simulink model "teste_amortecedor"  (R2019b)
settings: Solver=FixedStepAuto  StartTime=0.0  StopTime=10  FixedStep=10^-3  RelTol=1e-3
undefined symbols (not defined in the file or in its folder): sigbuilder_block
settings Model: Creator=aluno  LastModifiedBy=aluno

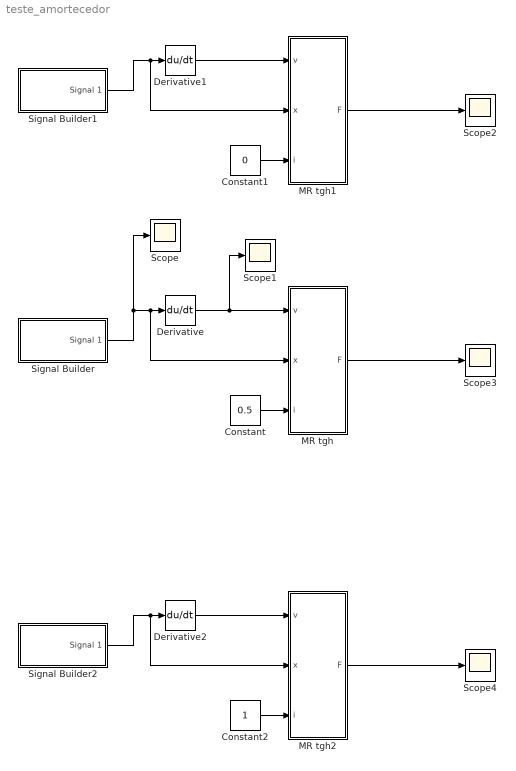
== system teste_amortecedor ==
  Constant : Constant  Value=0.5
  Constant1 : Constant  Value=0
  Constant2 : Constant
  Derivative : Derivative
  Derivative1 : Derivative
  Derivative2 : Derivative
  MR tgh : MATLAB Function  TreatAsAtomicUnit=on
  MR tgh1 : MATLAB Function  TreatAsAtomicUnit=on
  MR tgh2 : MATLAB Function  TreatAsAtomicUnit=on
  Scope{,1..4} (5 alike) : Scope
  Signal Builder : Subsystem  Tag=STV Subsys  LoadFcn=sigbuilder_block('load');  StartFcn=sigbuilder_block('start');  StopFcn=sigbuilder_block('stop');  ClipboardFcn=sigbuilder_block('clipboard');  mask(Sigbuilder block){tuvar=[0:10]}
      mask help: Simulink:masks:SigbuilderBlock_MD
      mask init:
      | if ~strcmp(get_param(bdroot(gcbh),'SimulationStatus'),'stopped') tuvar = sigbuilder_block('maskInit'); end
      settings: CopyFcn=sigbuilder_block('copy');  DeleteFcn=sigbuilder_block('delete');  ModelCloseFcn=sigbuilder_block('modelClose');  PreSaveFcn=sigbuilder_block('preSave');  PauseFcn=sigbuilder_block('pause');  ContinueFcn=sigbuilder_block('continue');  NameChangeFcn=sigbuilder_block('namechange');  OpenFcn=sigbuilder_block('open',[437.6 199.2 550.4 400 ]);  CloseFcn=sigbuilder_block('close');
      mask Display: plot(0, 0, 100, 100,[2, 2, 32, 32, 2], [68, 8, 8, 68, 68],[32, 2], [38, 38], [32, 19, 2],[53, 60, 44], [32, 17, 17, 2],[16, 16, 31, 31]);txt = getActiveGroup(gcbh);text(2, 100, txt,'verticalAlignment', 'top');
  Signal Builder1 : Subsystem  Tag=STV Subsys  LoadFcn=sigbuilder_block('load');  StartFcn=sigbuilder_block('start');  StopFcn=sigbuilder_block('stop');  ClipboardFcn=sigbuilder_block('clipboard');  mask(Sigbuilder block){tuvar=[0:10]}
      mask help: Simulink:masks:SigbuilderBlock_MD
      mask init:
      | if ~strcmp(get_param(bdroot(gcbh),'SimulationStatus'),'stopped') tuvar = sigbuilder_block('maskInit'); end
      settings: CopyFcn=sigbuilder_block('copy');  DeleteFcn=sigbuilder_block('delete');  ModelCloseFcn=sigbuilder_block('modelClose');  PreSaveFcn=sigbuilder_block('preSave');  PauseFcn=sigbuilder_block('pause');  ContinueFcn=sigbuilder_block('continue');  NameChangeFcn=sigbuilder_block('namechange');  OpenFcn=sigbuilder_block('open',[437.6 199.2 550.4 400 ]);  CloseFcn=sigbuilder_block('close');
      mask Display: plot(0, 0, 100, 100,[2, 2, 32, 32, 2], [68, 8, 8, 68, 68],[32, 2], [38, 38], [32, 19, 2],[53, 60, 44], [32, 17, 17, 2],[16, 16, 31, 31]);txt = getActiveGroup(gcbh);text(2, 100, txt,'verticalAlignment', 'top');
  Signal Builder2 : Subsystem  Tag=STV Subsys  LoadFcn=sigbuilder_block('load');  StartFcn=sigbuilder_block('start');  StopFcn=sigbuilder_block('stop');  ClipboardFcn=sigbuilder_block('clipboard');  mask(Sigbuilder block){tuvar=[0:10]}
      mask help: Simulink:masks:SigbuilderBlock_MD
      mask init:
      | if ~strcmp(get_param(bdroot(gcbh),'SimulationStatus'),'stopped') tuvar = sigbuilder_block('maskInit'); end
      settings: CopyFcn=sigbuilder_block('copy');  DeleteFcn=sigbuilder_block('delete');  ModelCloseFcn=sigbuilder_block('modelClose');  PreSaveFcn=sigbuilder_block('preSave');  PauseFcn=sigbuilder_block('pause');  ContinueFcn=sigbuilder_block('continue');  NameChangeFcn=sigbuilder_block('namechange');  OpenFcn=sigbuilder_block('open',[437.6 199.2 550.4 400 ]);  CloseFcn=sigbuilder_block('close');
      mask Display: plot(0, 0, 100, 100,[2, 2, 32, 32, 2], [68, 8, 8, 68, 68],[32, 2], [38, 38], [32, 19, 2],[53, 60, 44], [32, 17, 17, 2],[16, 16, 31, 31]);txt = getActiveGroup(gcbh);text(2, 100, txt,'verticalAlignment', 'top');
  wires:
  Constant/1 -> MR tgh/3(i)
  Signal Builder/1(Signal 1) -> Scope/1, MR tgh/2(x), Derivative/1
  Derivative/1 -> Scope1/1, MR tgh/1(v)
  MR tgh1/1(F) -> Scope2/1
  Constant1/1 -> MR tgh1/3(i)
  Signal Builder1/1(Signal 1) -> MR tgh1/2(x), Derivative1/1
  Derivative1/1 -> MR tgh1/1(v)
  Constant2/1 -> MR tgh2/3(i)
  Signal Builder2/1(Signal 1) -> MR tgh2/2(x), Derivative2/1
  Derivative2/1 -> MR tgh2/1(v)
  MR tgh/1(F) -> Scope3/1
  MR tgh2/1(F) -> Scope4/1

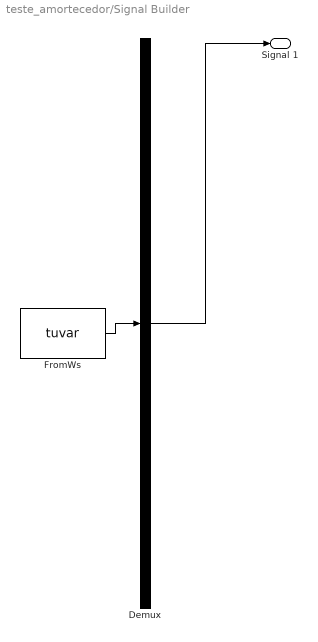
== system teste_amortecedor/Signal Builder ==
  Demux : Demux  Tag=STV Demux  Outputs=1
  FromWs : FromWorkspace  Tag=STV FromWs  VariableName=tuvar  SampleTime=0
      SigBuilderData=|
      | common.afterFinalStr = 'Extrapolate'
      | common.sampleTime = 0
      | dataSet.timeRange = [0 10]
      | dataSet.name = 'Group 1'
      | sbobj.Groups.Name = 'Group 1'
      | sbobj.Groups.Signals.Name = 'Signal 1'
      | sbobj.Groups.Signals.XData = [0 0.020202020202 0.040404040404 0.0606060606061 0.0808080808081 0.10101010101 0.121212121212 0.141414141414 0.161616161616 0.181818181818 0.20202020202 0.222222222222 ... (496 elements, 1x496)]
      | sbobj.Groups.Signals.YData = [0 0.000634239196566 0.00126592453574 0.0018925124436 0.00251147987181 0.00312033445698 0.0037166245566 0.00429794912089 0.004861967361 0.00540640817456 0.00592907929055 0.00642787609687 ... (496 elements, 1x496)]
  Signal 1 : Outport  Tag=STV Outport
  wires:
  Demux/1 -> Signal 1/1
  FromWs/1 -> Demux/1

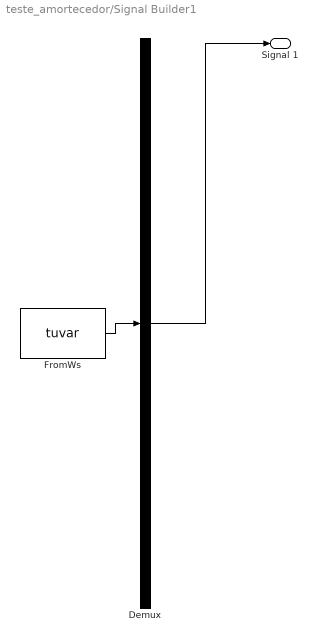
== system teste_amortecedor/Signal Builder1 ==
  Demux : Demux  Tag=STV Demux  Outputs=1
  FromWs : FromWorkspace  Tag=STV FromWs  VariableName=tuvar  SampleTime=0
      SigBuilderData=|
      | common.afterFinalStr = 'Extrapolate'
      | common.sampleTime = 0
      | dataSet.timeRange = [0 10]
      | dataSet.name = 'Group 1'
      | sbobj.Groups.Name = 'Group 1'
      | sbobj.Groups.Signals.Name = 'Signal 1'
      | sbobj.Groups.Signals.XData = [0 0.020202020202 0.040404040404 0.0606060606061 0.0808080808081 0.10101010101 0.121212121212 0.141414141414 0.161616161616 0.181818181818 0.20202020202 0.222222222222 ... (496 elements, 1x496)]
      | sbobj.Groups.Signals.YData = [0 0.000634239196566 0.00126592453574 0.0018925124436 0.00251147987181 0.00312033445698 0.0037166245566 0.00429794912089 0.004861967361 0.00540640817456 0.00592907929055 0.00642787609687 ... (496 elements, 1x496)]
  Signal 1 : Outport  Tag=STV Outport
  wires:
  Demux/1 -> Signal 1/1
  FromWs/1 -> Demux/1

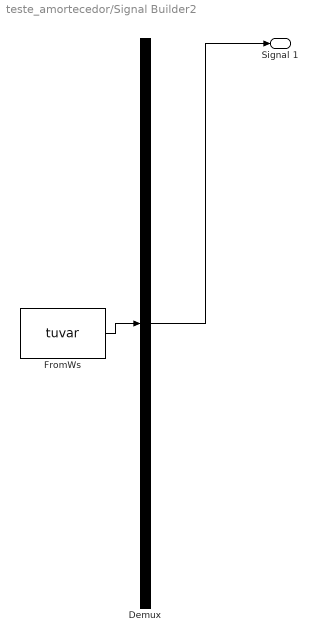
== system teste_amortecedor/Signal Builder2 ==
  Demux : Demux  Tag=STV Demux  Outputs=1
  FromWs : FromWorkspace  Tag=STV FromWs  VariableName=tuvar  SampleTime=0
      SigBuilderData=|
      | common.afterFinalStr = 'Extrapolate'
      | common.sampleTime = 0
      | dataSet.timeRange = [0 10]
      | dataSet.name = 'Group 1'
      | sbobj.Groups.Name = 'Group 1'
      | sbobj.Groups.Signals.Name = 'Signal 1'
      | sbobj.Groups.Signals.XData = [0 0.020202020202 0.040404040404 0.0606060606061 0.0808080808081 0.10101010101 0.121212121212 0.141414141414 0.161616161616 0.181818181818 0.20202020202 0.222222222222 ... (496 elements, 1x496)]
      | sbobj.Groups.Signals.YData = [0 0.000634239196566 0.00126592453574 0.0018925124436 0.00251147987181 0.00312033445698 0.0037166245566 0.00429794912089 0.004861967361 0.00540640817456 0.00592907929055 0.00642787609687 ... (496 elements, 1x496)]
  Signal 1 : Outport  Tag=STV Outport
  wires:
  Demux/1 -> Signal 1/1
  FromWs/1 -> Demux/1

== matlab function teste_amortecedor/MR tgh1 ==
  data: v input; x input; F output; i input
function F = tgh_model(v,x,i)
c = 1929*i+3200;
% k = -1700*i+5100;
k=0;
alpha = -244*i^2+918*i+32;
beta = 100;
delta = 0;
% f0 = -18*i-257;
f0=0;

F = k*x+c*v+alpha*tanh(beta*v+delta*sign(x))+f0;

== matlab function teste_amortecedor/MR tgh2 ==
  data: v input; x input; F output; i input
function F = tgh_model(v,x,i)
c = 1929*i+3200;
% k = -1700*i+5100;
k=0;
alpha = -244*i^2+918*i+32;
beta = 100;
delta = 0;
% f0 = -18*i-257;
f0=0;

F = k*x+c*v+alpha*tanh(beta*v+delta*sign(x))+f0;

== matlab function teste_amortecedor/MR tgh ==
  data: v input; x input; F output; i input
function F = tgh_model(v,x,i)
c = 1929*i+3200;
% k = -1700*i+5100;
k=0;
alpha = -244*i^2+918*i+32;
beta = 100;
delta = 0;
% f0 = -18*i-257;
f0=0;

F = k*x+c*v+alpha*tanh(beta*v+delta*sign(x))+f0;
